simulink model "system_input"  (R2020a)
settings: Solver=FixedStepAuto  StartTime=0.0  StopTime=95  FixedStep=0.05  RelTol=1e-3
libraries: simulink x1
settings Model: Creator=zeiph  LastModifiedBy=zeiph
settings DebuggingCC: ArithmeticOperatorsInVariantConditions=warning
settings SFSimCC: CustomCodeUndefinedFunction=UseInterfaceOnly

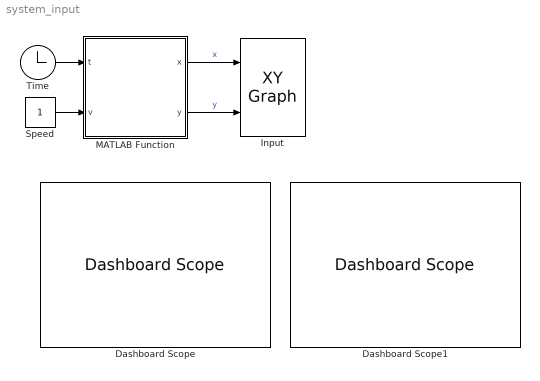
== system system_input ==
  Dashboard Scope : DashboardScope
  Dashboard Scope1 : DashboardScope
  Input : simulink/Sinks/XY Graph  xmin=-0.1  xmax=5.5  ymin=-5  ymax=13  st=-1
  MATLAB Function : MATLAB Function  TreatAsAtomicUnit=on
  Speed : Constant
  Time : Clock
  wires:
  Time/1 -> MATLAB Function/1(t)
  MATLAB Function/1(x) -> Input/1  "x"
  MATLAB Function/2(y) -> Input/2  "y"
  Speed/1 -> MATLAB Function/2(v)

== matlab function system_input/MATLAB Function ==
  data: x output; t input; y output; v input
function [x , y] = input(t , v)

    h = 10; %Straight line distance
    d = 5; %"Circle" diameter

    
    t = (mod(t , 2*h/v + 2*(d/v))); %% Loop

    is_on_part_1_flag = (t <= h/v);
    is_on_part_2_flag = (t > h/v && t <= h/v + d/v);
    is_on_part_3_flag = (t > h/v + d/v && t <= (2*h/v)+d/v); 
    is_on_part_4_flag = (~is_on_part_1_flag &&...
                         ~is_on_part_2_flag &&...
                         ~is_on_part_3_flag);
    
    timestamp = (is_on_part_1_flag) * t +...
                (is_on_part_2_flag) * (t - h/v) + ... 
                (is_on_part_3_flag) * (t - h/v - d/v)+...
                (is_on_part_4_flag) * (t - (2*h/v + (d/v)));


    y = is_on_part_1_flag * (timestamp*v)+...
        is_on_part_2_flag * (h + (d/2) * sin(pi*timestamp*v/d))+... 
        is_on_part_3_flag * (h-timestamp*v)+...
        is_on_part_4_flag * (-(d/2) * sin(pi*timestamp*v/d));

        
    x = is_on_part_1_flag * (0)+...
        is_on_part_2_flag * (timestamp*v)+... 
        is_on_part_3_flag * (d)+...
        is_on_part_4_flag * ((d - timestamp*v >0)*(d - timestamp*v));

            
            


end
